simulink model "suspension_statespace_r2019a"  (R2019a)
settings: Solver=VariableStepAuto  StartTime=0.0  StopTime=10.0  RelTol=1e-3
undefined symbols (not defined in the file): A, B, C, D
settings Model: Creator=byronmason  LastModifiedBy=byronmason
settings DataIOCC: Refine=10

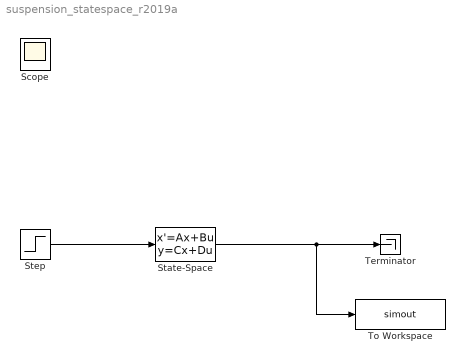
== system suspension_statespace_r2019a ==
  State-Space : StateSpace  A=A  B=B  C=C  D=D  InitialCondition=0
  Step : Step  Time=2  After=0.05  SampleTime=0
  Terminator : Terminator
  To Workspace : ToWorkspace  VariableName=simout  SampleTime=-1
  Scope : Scope
  wires:
  Step/1 -> State-Space/1
  State-Space/1 -> To Workspace/1, Terminator/1
